simulink model "max31855_task"  (Simulink 3.00)
libraries: mathlib x3, speclib x1, arclib x1

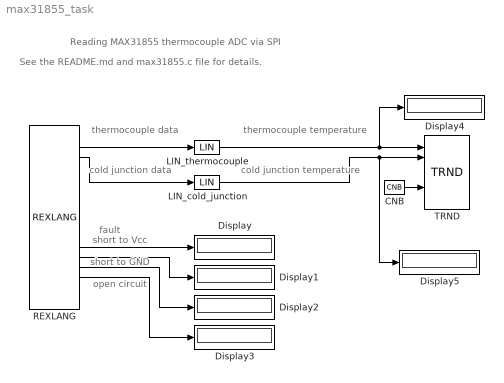
== system max31855_task ==
  note: Reading MAX31855 thermocouple ADC via SPI
  note: thermocouple data
  note: thermocouple temperature
  note: cold junction
      | data
  note: cold junction
      | temperature
  note: fault
  note: short to Vcc
  note: open circuit
  note: short to GND
  note: See the README.md and max31855.c file for details.
  CNB : mathlib/CNB  YCN=on
  Display{,1..5} (6 alike) : Display
      settings: Format=Best fit
  LIN_cold_junction : mathlib/LIN  u1=2032  y1=127  u2=-880  y2=-55
  LIN_thermocouple : mathlib/LIN  u1=6400  y1=1600  u2=-1000  y2=-250
  REXLANG : speclib/REXLANG  strs=0  SystemSampleTime=-1  tab_matlab=BASIC  srcname=max31855.c  srctype=1: C-like  stack=0  debug=3: Full check  p0=/dev/spidev0.0  p1=0  p2=0  p3=0  p4=0  p5=0  p6=0  p7=0  p8=0  p9=0  p10=0  p11=0  p12=0  p13=0  p14=0  p15=0  fname=/dev/spidev0.0
  TRND : arclib/TRND  n=4  l=1000  btype=8: Double  ptype1=1: Store  ptype2=1: Store  ptype3=1: Store  ptype4=1: Store  pfac=1  afac=0  arc=0  id=1  Title=Measured values  timesrc=1
  wires:
  CNB/1 -> TRND/5
  LIN_cold_junction/1 -> Display5/1, TRND/2
  LIN_thermocouple/1 -> Display4/1, TRND/1
  REXLANG/2 -> LIN_thermocouple/1
  REXLANG/3 -> LIN_cold_junction/1
  REXLANG/12 -> Display/1
  REXLANG/13 -> Display1/1
  REXLANG/14 -> Display2/1
  REXLANG/15 -> Display3/1
